simulink model "BungeeModelOld"  (R2024a)
settings: Solver=VariableStepAuto  StartTime=0.0  StopTime=10.0  RelTol=1e-3
undefined symbols (not defined in the file): c, g, k, L0, m, y0
settings Model: Creator=Daniel  LastModifiedBy=Daniel

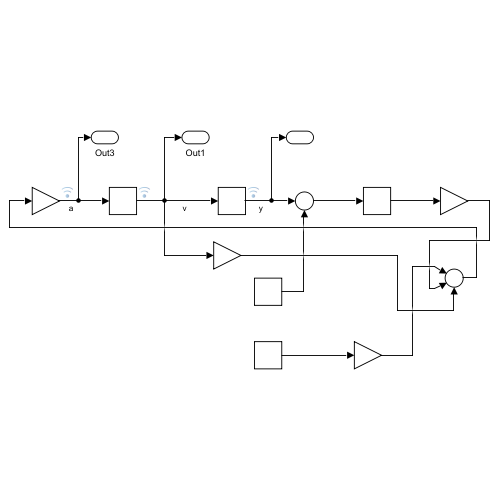
[thumbnail: Simulink's stored preview of the top-level diagram]
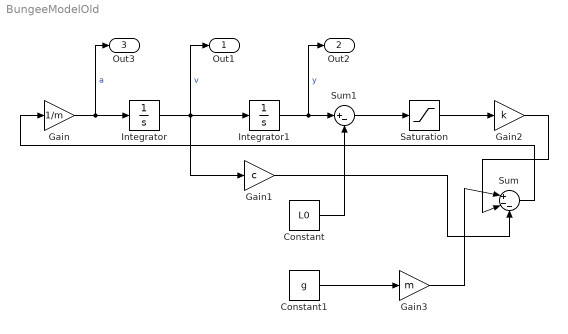
== system BungeeModelOld ==
  Constant : Constant  Value=L0
  Constant1 : Constant  Value=g
  Gain : Gain  Gain=1/m
  Gain1 : Gain  Gain=c
  Gain2 : Gain  Gain=k
  Gain3 : Gain  Gain=m
  Integrator : Integrator
  Integrator1 : Integrator  InitialCondition=y0
  Saturation : Saturate  UpperLimit=inf  LowerLimit=0
  Sum : Sum  Inputs=|+--
  Sum1 : Sum  Inputs=|+-
  Out1 : Outport
  Out2 : Outport  Port=2
  Out3 : Outport  Port=3
  wires:
  Gain/1 -> Out3/1, Integrator/1  "a"
  Integrator/1 -> Out1/1, Gain1/1, Integrator1/1  "v"
  Integrator1/1 -> Out2/1, Sum1/1  "y"
  Constant/1 -> Sum1/2
  Sum1/1 -> Saturation/1
  Saturation/1 -> Gain2/1
  Constant1/1 -> Gain3/1
  Gain3/1 -> Sum/1
  Gain2/1 -> Sum/2
  Gain1/1 -> Sum/3
  Sum/1 -> Gain/1
